simulink library "clq2pressuredropcoeff"  (R2018b)
settings: Solver=ode45  StartTime=0.0  StopTime=10.0  RelTol=1e-3  EnableMultiTasking=on
libraries: carnot x1
settings Model: Creator=lena.frank  LastModifiedBy=P41573
settings DataIOCC: LimitDataPoints=on  SaveFormat=Array  SignalLoggingSaveFormat=ModelDataLogs
settings OptimizationCC: ExpressionDepthLimit=2147483647  LifeSpan=inf
settings DebuggingCC: UnderspecifiedInitializationDetection=Classic  MergeDetectMultiDrivingBlocksExec=none  SolverPrmCheckMsg=warning  FcnCallInpInsideContextMsg=warning  StateNameClashWarn=warning  SFUnexpectedBacktrackingDiag=warning  SFNoUnconditionalDefaultTransitionDiag=warning  SFExecutionAtInitializationDiag=none
settings HardwareCC: ProdBitPerPointer=32  ProdBitPerSizeT=32  ProdBitPerPtrDiffT=32  ProdLargestAtomicFloat=None  ProdIntDivRoundTo=Undefined  ProdEndianess=Unspecified  ProdWordSize=32  ProdHWDeviceType=32-bit Generic
settings ModelReferenceCC: PropagateSignalLabelsOutOfModel=off
settings SFSimCC: SimUseLocalCustomCode=off
settings RTWCC: RTWUseLocalCustomCode=off
settings CodeAppCC: StateflowObjectComments=on
settings GRTTargetCC: TargetLangStandard=C89/C90 (ANSI)  GeneratePreprocessorConditionals=Disable all  CombineOutputUpdateFcns=off  GRTInterface=on
settings ConfigComp: CovMetricSettings=dw  CovHtmlReporting=on  CovSaveCumulativeToWorkspaceVar=on  CovSaveSingleToWorkspaceVar=on  CovExternalEMLEnable=off

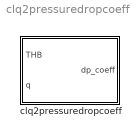
== system clq2pressuredropcoeff ==
  clq2pressuredropcoeff : Subsystem  mask(pressure drop coefficient 2 clq){}
      mask help:
      | Calculate the clq coefficients from the pressure drop coefficients.
      | dp = zeta * density/2 * w^2
      | dp = c + l*mdot + q*mdot^2    Carnot approach (here c = l = 0)
      | with mdot = Vdot*density = w*A*density  -> w = mdot/A/density
      | dp = zeta * density/2 * mdot^2/A^2/density^2
      | dp = zeta/(2*A^2*density) * mdot^2
      | -> q = zeta/(2*A^2*density)
      | with A = pi/4*d^2
      | -> q = 8*zeta / (pi^2*d^4*density)

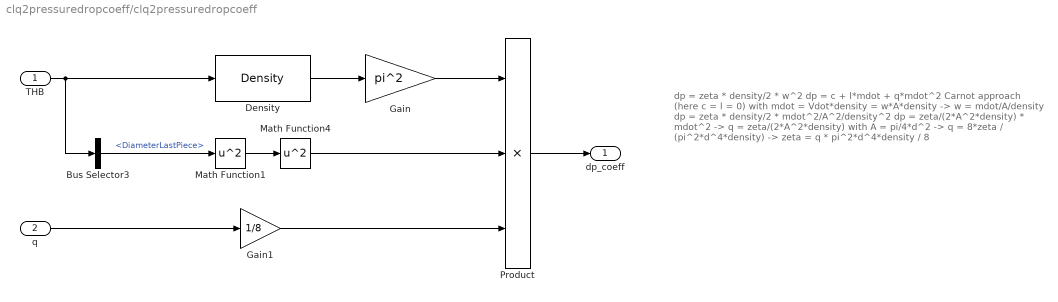
== system clq2pressuredropcoeff/clq2pressuredropcoeff ==
  note: dp = zeta * density/2 * w^2
      | dp = c + l*mdot + q*mdot^2    Carnot approach (here c = l = 0)
      | with mdot = Vdot*density = w*A*density  -> w = mdot/A/density
      | dp = zeta * density/2 * mdot^2/A^2/density^2
      | dp = zeta/(2*A^2*density) * mdot^2
      | -> q = zeta/(2*A^2*density)
      | with A = pi/4*d^2
      | -> q = 8*zeta / (pi^2*d^4*density)
      | -> zeta = q * pi^2*d^4*density / 8
  THB : Inport
  q : Inport  Port=2
  Bus Selector3 : BusSelector  OutputSignals=DiameterLastPiece
  Density : carnot/Basic/Material_Properties/Density  VariantControl=CarlibClassic  INPUTARGUMENTS=THB  DEBUGLEVEL=DEBUGLEVEL  MAXTOTALWARNINGS=inf  MAXCONSECUTIVEWARNINGS=inf  WRITETOFILE=0  FILENAME='errors.txt'
      settings: SourceProductName=Carnot
  Gain : Gain  Gain=pi^2
  Gain1 : Gain  Gain=1/8
  Math Function1 : Math  Operator=square  SaturateOnIntegerOverflow=on
  Math Function4 : Math  Operator=square  SaturateOnIntegerOverflow=on
  Product : Product  Inputs=3  RndMeth=Zero
  dp_coeff : Outport
  wires:
  Gain1/1 -> Product/3
  q/1 -> Gain1/1
  Math Function4/1 -> Product/2
  Math Function1/1 -> Math Function4/1
  Bus Selector3/1 -> Math Function1/1  "<DiameterLastPiece>"
  Density/1 -> Gain/1
  THB/1 -> Bus Selector3/1, Density/1
  Gain/1 -> Product/1
  Product/1 -> dp_coeff/1
